simulink model "Pizano_Lab10_Step1"  (R2016a)
settings: Solver=FixedStepDiscrete  StartTime=0.0  StopTime=30.0  FixedStep=.1  RelTol=1e-3
undefined symbols (not defined in the file): magnitude
libraries: simulink x1
settings Model: ModifiedComment=GODenergy -- Sun Dec 11 16:57:28 2016 -- Version 1.4  Creator=apizano  LastModifiedBy=GODenergy
settings Model: ModifiedHistory=|
  | GODenergy -- Sun Dec 11 16:57:28 2016 -- Version 1.4
  | 
  | 
  | GODenergy -- Sun Dec 11 16:56:54 2016 -- Version 1.3
  | 
  | 
  | GODenergy -- Sun Dec 11 16:56:00 2016 -- Version 1.2

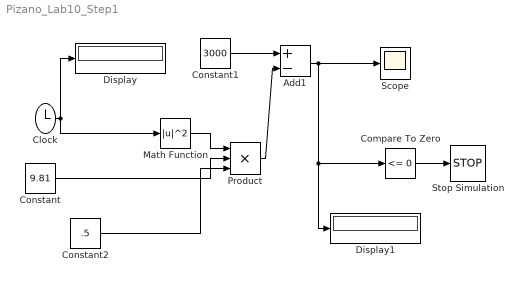
== system Pizano_Lab10_Step1 ==
  Add1 : Sum  Inputs=+-
  Clock : Clock
  Compare To Zero : simulink/Logic and Bit Operations/Compare To Zero  relop=<=  OutDataTypeStr=boolean
  Constant : Constant  Value=9.81
  Constant1 : Constant  Value=3000
  Constant2 : Constant  Value=.5
  Display : Display
  Display1 : Display
  Math Function : Math  Operator=magnitude^2  SaturateOnIntegerOverflow=on
  Product : Product  Inputs=3
  Scope : Scope
  Stop Simulation : Stop
  wires:
  Constant1/1 -> Add1/1
  Clock/1 -> Math Function/1, Display/1
  Math Function/1 -> Product/1
  Constant/1 -> Product/2
  Constant2/1 -> Product/3
  Product/1 -> Add1/2
  Add1/1 -> Compare To Zero/1, Display1/1, Scope/1
  Compare To Zero/1 -> Stop Simulation/1
